simulink model "Hybrid_P2_Parallel_ETE"  (R2017b)
settings: Solver=FixedStepAuto  StartTime=0.0  StopTime=length(Speed)  FixedStep=0.01  MaxStep=0.01  RelTol=1e-3  EnableMultiTasking=on
PostLoadFcn:
  | , if any(exist('dsrtsu_mdlpostloadfcn', 'file') == [2, 3, 6]), try dsrtsu_mdlpostloadfcn('Execute', bdroot); catch fprintf('Error in PostLoadFcn (dsrtsu_mdlpostloadfcn) for model "%s":\n %s\n', bdroot, lasterr); end, end,
undefined symbols (not defined in the file): Actuators, APP1_OOR, APP2_OOR, APP_Mismatch, Brk_Flt, cal, ClutchEngag, CycLength, CycNmb, DiscIntNeverNeededParam, eng, Engine, EngOverTemp, ENGTRQ_MSMCH_Degraded_CP, ENGTRQ_MSMCH_ErrCritical_CP, ENGTRQ_MSMCH_LimpHome_CP, EngTrqMismatch, ess, ESSOverTemp, gb, Gearbox, KeyPos_Flt, lib_Actuators, lib_EMachine_2017a, lib_Sensors_2017a, Loss, LossCAN, Machine, MCUOverTemp, mot, MotDirMismatch, MotOverTemp, MotTrqMismatch, PRNDL_Flt, Ratio, RegenFault, Scope_new, Scopes1, Sensors, Spd, StopIndex, t_amb, time, tloop
libraries: simulink x117, EC2_libraries x9, powerlib_meascontrol x2, CalculationGallon x1, lib_Chassis x1, lib_DCDC x1, lib_Differential x1, lib_HVESS x1, lib_Engine x1, lib_OBC x1, lib_Transmission x1, Transmission_Validation x1
(part 10 of 10)

== stateflow chart Hybrid_P2_Parallel_ETE/Controller_with_Transmission_Manager1/HSC/Powertrain Manager/Torque Distribution1/Supervisory  Control  Logic1 ==
  note: 
  state VehOn
    en:
    mode = 6;
    powerMode = 1;
    HV_Req=1;
  state VehOffOrAcc
    en:
    mode=0;
    powerMode = 0;
    EnablePrplsn = 0;
    HV_Req=0;
    closeMaincReq=0;
  note: Tranmission Shift Level Position (ShftLvrPos):
  state Close_Contactors
    en:
    closeMaincReq = 1;
  state ChgTrans
    en:
  state Wait1
  state VehShutdown
    en:
    powerMode = 1;
    EnablePrplsn = 0;
    EngOnReq = 0;
    EngAppReq = 0;
    EnableInverter=0;
    mode=8;
  state EnablePropulsion
    en:
    mode=7;
    EnablePrplsn = 1;
  note: System Power Mode (KeyPos):
  state Charging
    en:
    mode = 9;
    powerMode = 3;
    closeMaincReq = 1;
    EnablePrplsn = 0;
    EnableInverter = 0;
  state HV_Shutdown
    en:
    HV_Req=0;
    closeMaincReq=0;
  state IMG_Shutdown
    en:
    MotTrqReq = 0;
  state VehReady
    en:
    powerMode = 2;
    state Eng_Charging_NoReg [commented out]
      en:
      EngOnReq = 1;
      mode=2;
      du:
      MotTrqReq = MotTrqCalc(ShftLvrPos,DrvIntdAxleTrq,EngTrq,SoC,Voltage);
      EngTrq = EngTrqCalc(drvAPP,EngSpd,ShftLvrPos,DrvIntdAxleTrq,TransRatio);
      EngAppReq=drvAPP;
      state Trq = EngTrqCalc(EngSpeed,APP,ShftLvrPos,DrvIntdAxleTrq,TransRatio) [function] [commented out]
      state MotTrq = MotTrqCalc(ShftLvrPos,DrvIntdAxleTrq,Trq,SoC,Volt) [function] [commented out]
      state APP = EngTrq2EngApp(Trq,TransRatio) [function] [commented out]
    state Eng_Charging_Stat
      en:
      EngOnReq = 1;
      mode=5;
      du:
      MotTrqReq = MotTrqCalc(ShftLvrPos,DrvIntdAxleTrq,EngTrq,SoC,Voltage,drvAPP);
      EngTrq = EngTrqCalc(EngSpd,ShftLvrPos,DrvIntdAxleTrq,TransRatio);
      EngAppReq=drvAPP;
      state Trq = EngTrqCalc(EngSpeed,ShftLvrPos,DrvIntdAxleTrq,TransRatio) [function]
      state MotTrq = MotTrqCalc(ShftLvrPos,DrvIntdAxleTrq,Trq,SoC,Volt,APP) [function]
      state APP = EngTrq2EngApp(Trq,TransRatio) [function]
    state EnableINV
      en:
      EnableInverter = 1;
    state EnableINV2
      en:
      EnableInverter = 1;
    state CD_Mode
      en:
      mode=1;
      EngOnReq = 0;
      EngAppReq = 0;
      state Drive_mode
        en:
        Brkmode=0;
        du:
        MotTrqReq = MotTrqCalc2(drvAPP,ShftLvrPos,DrvIntdAxleTrq,TransRatio);
        state MotTrq = MotTrqCalc2(APP,ShftLvrPos,DrvIntdAxleTrq,TransRatio) [function]
      state Brake_mode
        en:
        EngAppReq=0;
        state Regen_mode
          en:
          Brkmode=1;
          du:
          MotTrqReq=MotTrqCalc1(BrkPdlPos,VehicleSpeed,...
          ShftLvrPos,MotSpd,TransRatio,IntdAxleTrq);
        state No_regen
          en:
          Brkmode=2;
          du:
          MotTrqReq=MotTrqCalc2(ShftLvrPos,TransRatio);
        state Temp_delay
        state Temp_delay1
        state T = MotTrqCalc1(BPP,VehSpd,ShftLvrPos,MotSpeed,TransRatio,IntdAxleTrq) [function]
        state T = MotTrqCalc2(ShftLvrPos,TransRatio) [function]
        (default) -> VehReady.CD_Mode.Brake_mode.No_regen
        VehReady.CD_Mode.Brake_mode.Regen_mode -> VehReady.CD_Mode.Brake_mode.Temp_delay : [RegenBrkDisable||SoC>=80||ABSAtv||Regen_fault]
        VehReady.CD_Mode.Brake_mode.Temp_delay -> VehReady.CD_Mode.Brake_mode.No_regen : after(0.25,sec)
        VehReady.CD_Mode.Brake_mode.Temp_delay1 -> VehReady.CD_Mode.Brake_mode.Regen_mode : after(0.25,sec)
        VehReady.CD_Mode.Brake_mode.No_regen -> VehReady.CD_Mode.Brake_mode.Temp_delay1 : [RegenBrkDisable == 0&&SoC<80&&ABSAtv==0&&Regen_fault==0]
      state Time_delay
      state Time_delay1
      (default) -> Drive_mode
      Drive_mode -> Time_delay : [BrkPdlPos>0&&IntdAxleTrq<0]
      Time_delay -> Brake_mode : after(0.25,sec)
      Time_delay1 -> Drive_mode : after(0.25,sec)
      Brake_mode -> Time_delay1 : [drvAPP>0&&IntdAxleTrq>=0]
    state EnableINV1
      en:
      EnableInverter = 1;
    state Engine_Charge
      en:
      mode=2;
      EngOnReq=1;
      state Eng_Charge_CS
        en:
        Brkmode=0;
        du:
        MotTrqReq = MotTrqCalc(ShftLvrPos,DrvIntdAxleTrq,EngTrq,SoC,Voltage);
        EngTrq = EngTrqCalc(drvAPP,EngSpd,ShftLvrPos,DrvIntdAxleTrq,TransRatio);
        EngAppReq=EngTrq2EngApp(EngTrq,TransRatio);
        state Trq = EngTrqCalc(EngSpeed,APP,ShftLvrPos,DrvIntdAxleTrq,TransRatio) [function]
        state MotTrq = MotTrqCalc(ShftLvrPos,DrvIntdAxleTrq,Trq,SoC,Volt) [function]
        state APP = EngTrq2EngApp(Trq,TransRatio) [function]
      state Brake_mode1
        en:
        EngAppReq=0.51;
        state Regen_mode
          en:
          Brkmode=1;
          du:
          MotTrqReq=MotTrqCalc1(BrkPdlPos,VehicleSpeed,...
          ShftLvrPos,MotSpd,TransRatio,IntdAxleTrq);
        state No_regen
          en:
          Brkmode=2;
          du:
          MotTrqReq=MotTrqCalc2(ShftLvrPos,TransRatio);
        state Temp_delay
        state Temp_delay1
        state T = MotTrqCalc1(BPP,VehSpd,ShftLvrPos,MotSpeed,TransRatio,IntdAxleTrq) [function]
        state T = MotTrqCalc2(ShftLvrPos,TransRatio) [function]
        (default) -> VehReady.Engine_Charge.Brake_mode1.No_regen
        VehReady.Engine_Charge.Brake_mode1.Regen_mode -> VehReady.Engine_Charge.Brake_mode1.Temp_delay : [RegenBrkDisable||SoC>=80||ABSAtv||Regen_fault]
        VehReady.Engine_Charge.Brake_mode1.Temp_delay -> VehReady.Engine_Charge.Brake_mode1.No_regen : after(0.25,sec)
        VehReady.Engine_Charge.Brake_mode1.Temp_delay1 -> VehReady.Engine_Charge.Brake_mode1.Regen_mode : after(0.25,sec)
        VehReady.Engine_Charge.Brake_mode1.No_regen -> VehReady.Engine_Charge.Brake_mode1.Temp_delay1 : [RegenBrkDisable == 0&&EngSpd>1000&&SoC<80&&ABSAtv==0&&Regen_fault==0]
      state Time_delay3
      state Time_delay2
      (default) -> Eng_Charge_CS
      Eng_Charge_CS -> Time_delay3 : [BrkPdlPos>0 && IntdAxleTrq<0]
      Time_delay3 -> Brake_mode1 : after(0.25,sec)
      Time_delay2 -> Eng_Charge_CS : after(0.25,sec)
      Brake_mode1 -> Time_delay2 : [drvAPP>0&&IntdAxleTrq>=0]
    (default) -> (junction 1566)
    EnableINV2 -> Eng_Charging_Stat : [INV_State == 8]
    (junction 1566) -> EnableINV2 [order 3] : [!SW_CS_ON&&...
        | CDmode == 0&&SW_Engine_ON&&...
        | ShftLvrPos==1&&HoodStatus==0]
    (junction 1566) -> EnableINV [order 1] : [CDmode == 1 && !SW_Engine_ON&&...
        | !SW_CS_ON]
    EnableINV -> CD_Mode : [INV_State == 8]
    (junction 1566) -> EnableINV1 [order 2] : [SW_CS_ON&&...
        | CDmode == 0&&!SW_Engine_ON]
    EnableINV1 -> Engine_Charge : [INV_State == 8]
  VehOffOrAcc -> VehOn [order 1] : [KeyPos>= 1&&(eSystemStatus||iceSystemStatus)]
  VehOn -> VehOffOrAcc [order 2] : [KeyPos < 1]
  (default) -> VehOffOrAcc
  VehOn -> Close_Contactors [order 1] : [INV_State == 3]
  Close_Contactors -> VehOffOrAcc [order 2] : [KeyPos < 1]
  ChgTrans -> VehOffOrAcc [order 2] : [plugged==0]
  VehOffOrAcc -> ChgTrans [order 2] : [plugged]
      | {HV_Req=1;}
  (default) -> ? [commented out] : [KeyPos==3&&BrkPdlPos>10&&ShftLvrPos==1&&(~eSystemStatus&&iceSystemStatus)]
  VehShutdown -> VehOffOrAcc : after(1,sec)...
      | [plugged==0]
  Wait1 -> VehOffOrAcc [order 2] : after(3,sec)[plugged==0]
  ChgTrans -> Charging [order 1] : after(4,sec)...
      | [INV_State==3]
  Close_Contactors -> Charging [order 3] : [plugged]
  Close_Contactors -> EnablePropulsion [order 1] : [KeyPos==3&&BrkPdlPos>10&&...
      | ShftLvrPos==1&&IstModus==1]
  Charging -> Wait1 : [plugged==0]
  Wait1 -> Charging [order 1] : after(3,sec)[plugged==1]
  HV_Shutdown -> VehShutdown : [(INV_State==3||INV_State==14)]
  EnablePropulsion -> Charging [order 2] : [plugged]
  EnablePropulsion -> VehReady [order 1] : after(0.5,sec)
  IMG_Shutdown -> HV_Shutdown : [MotSpd<10&&ShftLvrPos==1]
  VehReady -> Charging [order 1] : [plugged]
  VehReady -> IMG_Shutdown [order 2] : [KeyPos < 2 ||(eSystemStatus==0&&iceSystemStatus==0)||SoC<10]
  data: Trq function_output double size=1; EngSpeed function_input double size=1; APP function_input double size=1; ShftLvrPos function_input double size=1; DrvIntdAxleTrq function_input double size=1; TransRatio function_input double size=1; MotTrq function_output double size=1; ShftLvrPos function_input double size=1; DrvIntdAxleTrq function_input double size=1; Trq function_input double size=1; SoC function_input double size=1; Volt function_input double size=1; Trq function_input double size=1; APP function_output double size=1; TransRatio function_input double size=1; Trq function_output; EngSpeed function_input; ShftLvrPos function_input; DrvIntdAxleTrq function_input; TransRatio function_input; MotTrq function_output; ShftLvrPos function_input; DrvIntdAxleTrq function_input; Trq function_input; SoC function_input; Volt function_input; APP function_input; Trq function_input; APP function_output; TransRatio function_input; APP function_input; MotTrq function_output; ShftLvrPos function_input; DrvIntdAxleTrq function_input; TransRatio function_input; T function_output; BPP function_input; VehSpd function_input; ShftLvrPos function_input; MotSpeed function_input; TransRatio function_input; IntdAxleTrq function_input; T function_output; ShftLvrPos function_input; TransRatio function_input; Trq function_output; EngSpeed function_input; APP function_input; ShftLvrPos function_input; DrvIntdAxleTrq function_input; TransRatio function_input; MotTrq function_output; ShftLvrPos function_input; DrvIntdAxleTrq function_input; Trq function_input; SoC function_input; Volt function_input; Trq function_input; APP function_output; TransRatio function_input; T function_output; BPP function_input; VehSpd function_input; ShftLvrPos function_input; MotSpeed function_input; TransRatio function_input; IntdAxleTrq function_input; T function_output; ShftLvrPos function_input; TransRatio function_input; TransEstGear input int8; SportModeEnabled input boolean; mode output int8; powerMode output int8; closeMaincReq output double; EnablePrplsn output boolean; KeyPos input int8; BrkPdlPos input double; drvAPP input double; VehicleSpeed input double; EngSpd input double; MotSpd input double; ShftLvrPos input int8; EngAppReq output double; EngOnReq output boolean; MotTrqReq output double; EnableInverter output boolean; InverterEnabled input double; plugged input double; CD_SOC_MIN input double; CS_SOC_MIN input double; CS_SOC_MAX input double; EngRunAtv input boolean; SoC input double; Voltage input double; EngTrq output double; DrvIntdAxleTrq input double; IntdAxleTrq input double; Faked_SoC input double; TransRatio input double; HV_Req output double; SW_CS_ON input boolean; SW_Engine_ON input; RegenBrkDisable input boolean; Chg output double; Brkmode output double; Drvmode output double; eSystemStatus input; iceSystemStatus input; Drv_Mode local double; ABSAtv input boolean; Regen_fault input boolean; EngFdbkTrq input double; EngCtlTmp input; CDmode input double; INV_State input; HoodStatus input; IstModus input

== stateflow chart Hybrid_P2_Parallel_ETE/Controller_with_Transmission_Manager1/HSC/Powertrain Manager/Torque Distribution1/Sports Mode Logic ==
  state Sport_Mode
    entry:
    Driver_Mode=2;
  state Hybrid_Mode
    entry:
    Driver_Mode=1;
  Hybrid_Mode -> Sport_Mode : [Voltage_Input>3.5&&Voltage_Input<3.9]
  (default) -> Hybrid_Mode
  Sport_Mode -> Hybrid_Mode : [Voltage_Input>1.8&&Voltage_Input<2.2]
  data: Voltage_Input input; Driver_Mode output

== stateflow chart Hybrid_P2_Parallel_ETE/Controller_with_Transmission_Manager1/HSC/Powertrain Manager/Thermal Manager/ESS Pump Manger/Chart1 ==
  state ESS_Pump [parallel]
    settings: executionOrder=1
    state pump_state_0
      entry: ESS_pump_control=0;
    state pump_low_State_1
      entry: ESS_pump_control=30;
    state pump_transition_3_to_0
    state pump_transition_2_to_0
    state pump_high_State_3
      entry: ESS_pump_control=90;
    state pump_medi_State_2
      entry: ESS_pump_control=60;
    pump_state_0 -> pump_low_State_1 : [(ESS_temp>=ESS_Temp_State_1_Thrs)&&SysPowMod>0]
    (default) -> pump_state_0
    pump_low_State_1 -> pump_state_0 [order 1] : [(ESS_temp<ESS_Temp_State_1_Thrs&&after(10,sec))||SysPowMod==0 ]
    pump_transition_2_to_0 -> pump_state_0 : after(15,sec)
    pump_transition_3_to_0 -> pump_state_0 : after(30,sec)
    pump_low_State_1 -> pump_medi_State_2 [order 2] : [ESS_temp>=ESS_Temp_State_2_Thrs]
    pump_medi_State_2 -> pump_low_State_1 [order 1] : [ESS_temp<ESS_Temp_State_2_Thrs&&after(10,sec)]
    pump_high_State_3 -> pump_transition_3_to_0 [order 2] : [SysPowMod==0]
    pump_medi_State_2 -> pump_transition_2_to_0 [order 3] : [SysPowMod==0]
    pump_medi_State_2 -> pump_high_State_3 [order 2] : [ESS_temp>=ESS_Temp_State_3_Thrs]
    pump_high_State_3 -> pump_medi_State_2 [order 1] : [ESS_temp<ESS_Temp_State_3_Thrs&&after(10,sec)]
  state ESS_comp [parallel]
    settings: executionOrder=2
    state Comp_off
      entry:
      ESS_comp=0;
      ESS_val=0;
      ESS_comp_Enable = 1;
    state Comp_on
      entry:
      ESS_comp=10;
      ESS_val=1;
      ESS_comp_Enable = 0;
    (default) -> Comp_off
    Comp_off -> Comp_on : [(ESS_CltTemp>=ESS_Comp_TempThrs)&&SysPowMod>0]
    Comp_on -> Comp_off : [(ESS_CltTemp<ESS_Comp_TempThrs&&after(25,sec))&&SysPowMod==0]
  data: ESS_temp input; ESS_comp output; ESS_pump_control output; ESS_val output; ESS_Temp_State_1_Thrs input double =15; ESS_Temp_State_2_Thrs input double; ESS_Temp_State_3_Thrs input double; ESS_Comp_TempThrs input double; ESS_CltTemp input; ESS_comp_Enable output; SysPowMod input

== stateflow chart Hybrid_P2_Parallel_ETE/Controller_with_Transmission_Manager1/HSC/Powertrain Manager/Thermal Manager/MotInv Pump Manger/MCUPump_Manager ==
  state Pump_Off
    entry: MotInvpump_control=0;
  state Pump_transition_2_to_off
  state Pump_High_State_2
    entry: MotInvpump_control=90;
  state Pump_Low_State_1
    entry: MotInvpump_control=60;
  (default) -> Pump_Off
  Pump_transition_2_to_off -> Pump_Off : after(30,sec)
  Pump_Off -> Pump_Low_State_1 : [(Motor_temp>=Mot_Temp_State_1_Thrs||MCU_temp>=MCU_Temp_State_1_Thrs)&&after(10,sec)&&SysPowMod>0]
  Pump_Low_State_1 -> Pump_Off [order 2] : [((Motor_temp<Mot_Temp_State_1_Thrs)&&(MCU_temp<MCU_Temp_State_1_Thrs)&&after(10,sec))||SysPowMod==0]
  Pump_High_State_2 -> Pump_transition_2_to_off [order 2] : [SysPowMod==0]
  Pump_Low_State_1 -> Pump_High_State_2 [order 1] : [(Motor_temp>=Mot_Temp_State_2_Thrs||MCU_temp>=MCU_Temp_State_2_Thrs)&&after(10,sec)]
  Pump_High_State_2 -> Pump_Low_State_1 [order 1] : [(Motor_temp<Mot_Temp_State_2_Thrs&&MCU_temp<MCU_Temp_State_2_Thrs)&&(after(10,sec))]
  data: MotInvpump_control output; Motor_temp input; MCU_temp input; MCU_Temp_State_1_Thrs input double; Mot_Temp_State_1_Thrs input double; MCU_Temp_State_2_Thrs input double; Mot_Temp_State_2_Thrs input double; SysPowMod input
